simulink model "CubeSat_SDP_PD_Attitude"  (R2024b)
settings: Solver=FixedStepAuto  StartTime=0.0  StopTime=T_total  FixedStep=delta_t  MaxStep=delta_t  MinStep=delta_t
values from neighbouring files (symbols this model uses):
  Cross_section_area = 0.01    [initialize_satellite_simulation.m]
  finalAttitude = finalAttitude/norm(finalAttitude)    [initialize_satellite_simulation.m]
  J = diag([Jxx, Jxx, Jxx])    [calculateInertiaTensor.m]    (also in initialize_satellite_simulation.m = calculateInertiaTensor(mass, sideLength); solveSDPControl.m = reshape(u(9:17), 3, 3))
  J2 = J(2,2)    [cvx_sdp.m]
  k_d = 0.02    [initialize_satellite_simulation.m]
  k_p = 1.0    (= 1)    [initialize_satellite_simulation.m]
  mass = 1.33    [initialize_satellite_simulation.m]
undefined symbols (not defined in the file or in its folder): compute_drag
libraries: aerolibutil x6, aerolibgravity2 x1
settings Model: PauseTimes=0.2  PacingRate=1.100000  VariantFading=off  LastModifiedBy=shavykashyap
settings SolverCC: InitialStep=delta_t  ZeroCrossAlgorithm=Adaptive
settings DataIOCC: Refine=2
settings DebuggingCC: SignalInfNanChecking=error  MaskedZcDiagnostic=none  IgnoredZcDiagnostic=none  CheckMatrixSingularityMsg=error

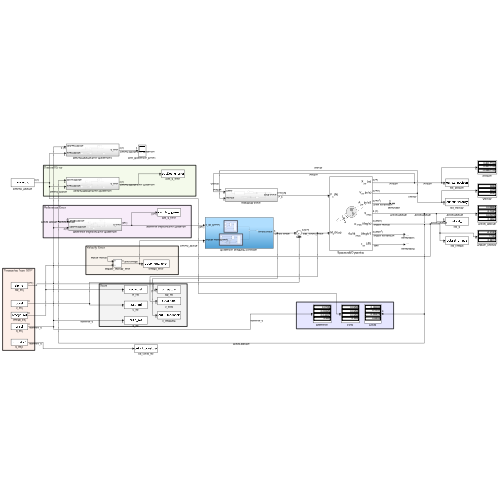
[thumbnail: Simulink's stored preview of the top-level diagram]
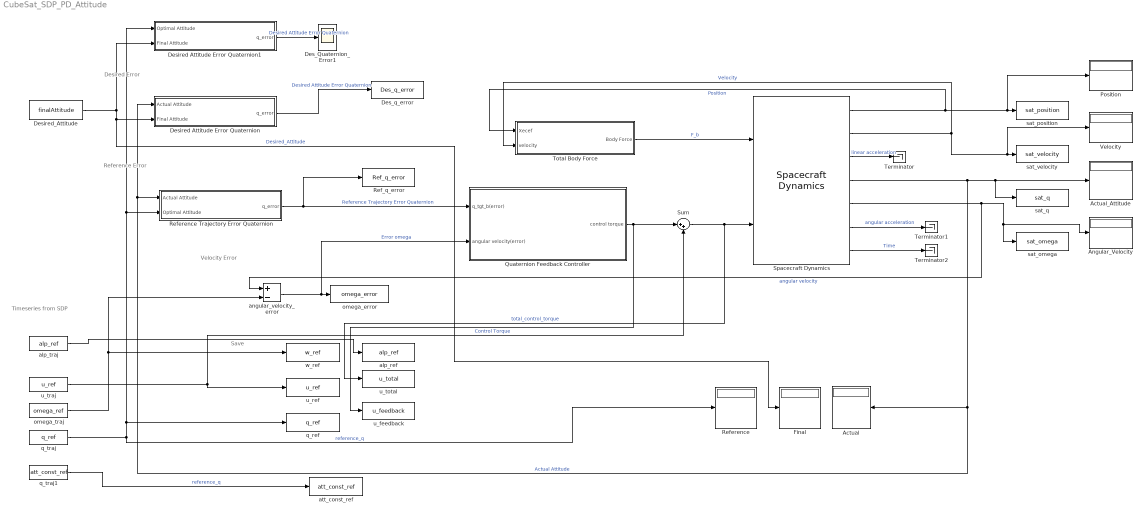
== system CubeSat_SDP_PD_Attitude ==
  note: Save
  note: Velocity Error
  note: Reference Error
  note: Timeseries from SDP
  note: Desired Error
  Actual : Display
  Actual_Attitude : Display
  "Angular_Velocity " : Display
  Des_Quaternion_Error1 : Scope
  Des_q_error : ToWorkspace  VariableName=Des_q_error  SaveFormat=Timeseries  SampleTime=-1
  Desired Attitude Error Quaternion : Subsystem
  Desired Attitude Error Quaternion1 : Subsystem
  Desired_Attitude : Constant  Value=finalAttitude
  Final : Display
  Position : Display
  "Quaternion Feedback Controller " : Subsystem
  Ref_q_error : ToWorkspace  VariableName=Ref_q_error  SaveFormat=Timeseries  SampleTime=-1
  Reference : Display
  Reference Trajectory Error Quaternion : Subsystem
  Spacecraft Dynamics : SpacecraftDynamics  outputAccel=on  mass=mass  inertia=J  stateFormatNum=ICRF state vector  inertialPosition=initialPosition  inertialVelocity=initialVelocity  attitude=initialAttitude  attitudeRate=initialAngularVelocity  outputAngAccel=on  gravityModel=Oblate ellipsoid (J2)  useDrag=on  useSRP=on
  Sum : Sum  Inputs=|++
  Terminator : Terminator
  Terminator1 : Terminator
  Terminator2 : Terminator
  "Total Body Force " : Subsystem
  Velocity : Display
  alp_ref : ToWorkspace  VariableName=alp_ref  SaveFormat=Timeseries  SampleTime=-1
  alp_traj : FromWorkspace  VariableName=alp_ref
  angular_velocity_error : Sum  Inputs=+-
  att_const_ref : ToWorkspace  VariableName=att_const_ref  SaveFormat=Timeseries  SampleTime=-1
  omega_error : ToWorkspace  VariableName=omega_error  SaveFormat=Timeseries  SampleTime=-1
  omega_traj : FromWorkspace  VariableName=omega_ref
  q_ref : ToWorkspace  VariableName=q_ref  SaveFormat=Timeseries  SampleTime=-1
  q_traj : FromWorkspace  VariableName=q_ref
  q_traj1 : FromWorkspace  VariableName=att_const_ref
  sat_omega : ToWorkspace  VariableName=sat_omega  SaveFormat=Timeseries  SampleTime=-1
  sat_position : ToWorkspace  VariableName=sat_position  SaveFormat=Timeseries  SampleTime=-1
  sat_q : ToWorkspace  VariableName=sat_q  SaveFormat=Timeseries  SampleTime=-1
  sat_velocity : ToWorkspace  VariableName=sat_velocity  SaveFormat=Timeseries  SampleTime=-1
  u_feedback : ToWorkspace  VariableName=u_feedback  SaveFormat=Timeseries  SampleTime=-1
  u_ref : ToWorkspace  VariableName=u_ref  SaveFormat=Timeseries  SampleTime=-1
  u_total : ToWorkspace  VariableName=u_total  SaveFormat=Timeseries  SampleTime=-1
  u_traj : FromWorkspace  VariableName=u_ref
  w_ref : ToWorkspace  VariableName=w_ref  SaveFormat=Timeseries  SampleTime=-1
  wires:
  Spacecraft Dynamics/1 -> "Total Body Force "/1(Xecef), Position/1, sat_position/1  "Position"
  Spacecraft Dynamics/2 -> Velocity/1, sat_velocity/1, "Total Body Force "/2(velocity)  "Velocity"
  Spacecraft Dynamics/4 -> Desired Attitude Error Quaternion/1(Actual Attitude), Reference Trajectory Error Quaternion/1(Actual Attitude), Actual/1, sat_q/1, Actual_Attitude/1  "Actual Attitude"
  Spacecraft Dynamics/5 -> angular_velocity_error/1, "Angular_Velocity "/1, sat_omega/1  "angular velocity"
  "Quaternion Feedback Controller "/1(control torque) -> Sum/1, u_feedback/1  "Control Torque"
  Desired_Attitude/1 -> Desired Attitude Error Quaternion/2(Final Attitude), Final/1, Desired Attitude Error Quaternion1/2(Final Attitude)  "Desired_Attitude"
  Spacecraft Dynamics/6 -> Terminator1/1  "angular acceleration"
  Spacecraft Dynamics/7 -> Terminator2/1  "Time"
  Spacecraft Dynamics/3 -> Terminator/1  "linear acceleration"
  "Total Body Force "/1(Body Force) -> Spacecraft Dynamics/1  "F_b"
  Sum/1 -> u_total/1, Spacecraft Dynamics/2  "total_control_torque"
  Reference Trajectory Error Quaternion/1(q_error) -> "Quaternion Feedback Controller "/1(q_tgt_b(error)), Ref_q_error/1  "Reference Trajectory Error Quaternion"
  angular_velocity_error/1 -> "Quaternion Feedback Controller "/2(angular velocity(error)), omega_error/1  "Error omega"
  Desired Attitude Error Quaternion/1(q_error) -> Des_q_error/1  "Desired Attitude Error Quaternion"
  u_traj/1 -> u_ref/1, Sum/2
  omega_traj/1 -> angular_velocity_error/2, w_ref/1
  q_traj/1 -> Reference/1, q_ref/1, Desired Attitude Error Quaternion1/1(Optimal Attitude), Reference Trajectory Error Quaternion/2(Optimal Attitude)  "reference_q"
  Desired Attitude Error Quaternion1/1(q_error) -> Des_Quaternion_Error1/1  "Desired Attitude Error Quaternion"
  alp_traj/1 -> alp_ref/1
  q_traj1/1 -> att_const_ref/1  "reference_q"

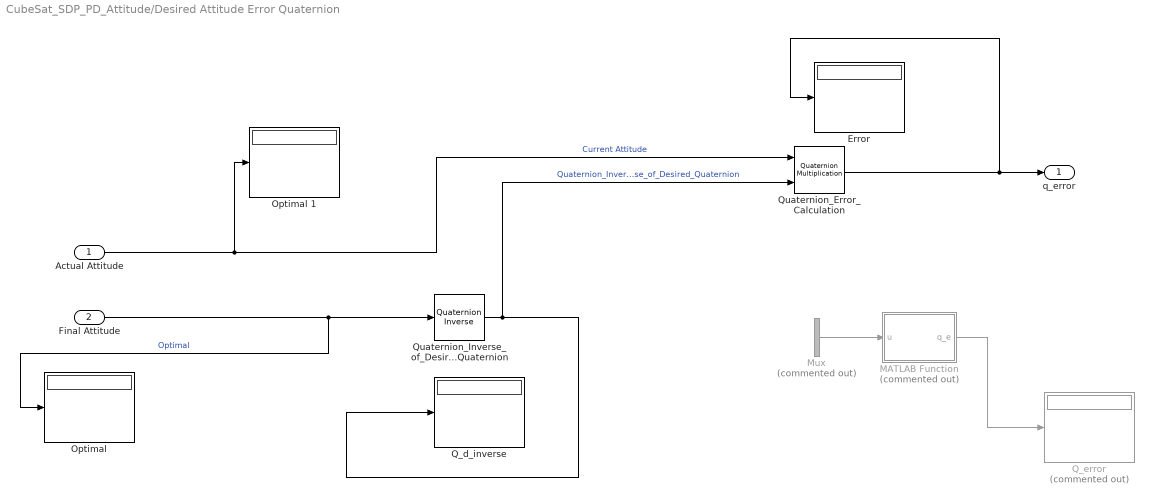
== system CubeSat_SDP_PD_Attitude/Desired Attitude Error Quaternion ==
  Actual Attitude : Inport
  Final Attitude : Inport  Port=2
  Error : Display
  MATLAB Function : MATLAB Function  Commented=on  TreatAsAtomicUnit=on
  Mux : Mux  Commented=on  Inputs=2
  "Optimal " : Display
  Optimal 1 : Display
  Q_d_inverse : Display
  Q_error : Display  Commented=on
  Quaternion_Error_Calculation : aerolibutil/Quaternion Multiplication
  Quaternion_Inverse_of_Desired_Quaternion : aerolibutil/Quaternion Inverse
  q_error : Outport
  wires:
  Actual Attitude/1 -> Optimal 1/1, Quaternion_Error_Calculation/1  "Current Attitude"
  Quaternion_Inverse_of_Desired_Quaternion/1 -> Quaternion_Error_Calculation/2, Q_d_inverse/1  "Quaternion_Inverse_of_Desired_Quaternion"
  Quaternion_Error_Calculation/1 -> q_error/1, Error/1
  Final Attitude/1 -> Quaternion_Inverse_of_Desired_Quaternion/1, "Optimal "/1  "Optimal"
  Mux/1 -> MATLAB Function/1(u)
  MATLAB Function/1(q_e) -> Q_error/1

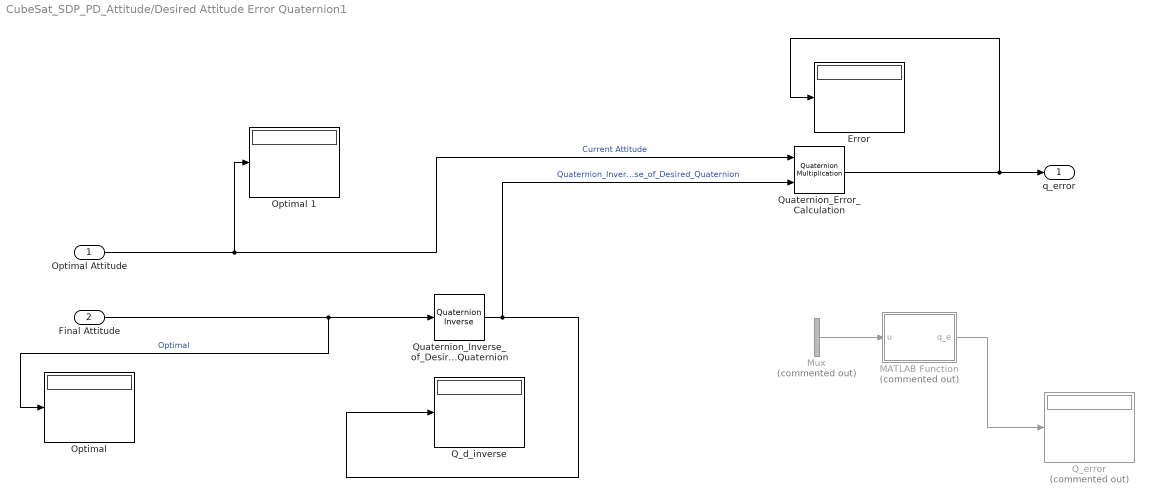
== system CubeSat_SDP_PD_Attitude/Desired Attitude Error Quaternion1 ==
  Optimal Attitude : Inport
  Final Attitude : Inport  Port=2
  Error : Display
  MATLAB Function : MATLAB Function  Commented=on  TreatAsAtomicUnit=on
  Mux : Mux  Commented=on  Inputs=2
  "Optimal " : Display
  Optimal 1 : Display
  Q_d_inverse : Display
  Q_error : Display  Commented=on
  Quaternion_Error_Calculation : aerolibutil/Quaternion Multiplication
  Quaternion_Inverse_of_Desired_Quaternion : aerolibutil/Quaternion Inverse
  q_error : Outport
  wires:
  Optimal Attitude/1 -> Optimal 1/1, Quaternion_Error_Calculation/1  "Current Attitude"
  Quaternion_Inverse_of_Desired_Quaternion/1 -> Quaternion_Error_Calculation/2, Q_d_inverse/1  "Quaternion_Inverse_of_Desired_Quaternion"
  Quaternion_Error_Calculation/1 -> q_error/1, Error/1
  Final Attitude/1 -> Quaternion_Inverse_of_Desired_Quaternion/1, "Optimal "/1  "Optimal"
  Mux/1 -> MATLAB Function/1(u)
  MATLAB Function/1(q_e) -> Q_error/1

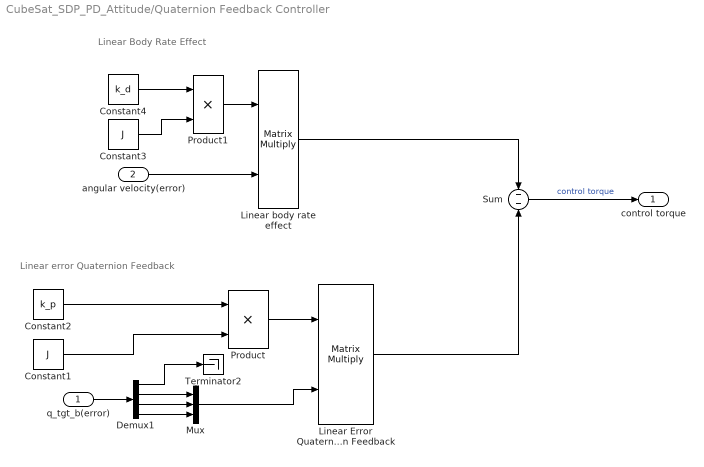
== system CubeSat_SDP_PD_Attitude/Quaternion Feedback Controller  ==
  note: Linear error Quaternion Feedback
  note: Linear Body Rate Effect
  q_tgt_b(error) : Inport
  angular velocity(error) : Inport  Port=2
  Constant1 : Constant  Value=J
  Constant2 : Constant  Value=k_p
  Constant3 : Constant  Value=J
  Constant4 : Constant  Value=k_d
  Demux1 : Demux
  Linear Error Quaternion Feedback : Product  Multiplication=Matrix(*)
  Linear body rate effect : Product  Multiplication=Matrix(*)
  Mux : Mux  Inputs=3
  Product : Product
  Product1 : Product
  Sum : Sum  Inputs=--
  Terminator2 : Terminator
  control torque : Outport
  wires:
  Linear body rate effect/1 -> Sum/1
  Mux/1 -> Linear Error Quaternion Feedback/2
  angular velocity(error)/1 -> Linear body rate effect/2
  Demux1/1 -> Terminator2/1
  Constant1/1 -> Product/2
  Linear Error Quaternion Feedback/1 -> Sum/2
  Demux1/4 -> Mux/3
  Constant2/1 -> Product/1
  Demux1/2 -> Mux/1
  Demux1/3 -> Mux/2
  Constant3/1 -> Product1/2
  q_tgt_b(error)/1 -> Demux1/1
  Sum/1 -> control torque/1  "control torque"
  Constant4/1 -> Product1/1
  Product/1 -> Linear Error Quaternion Feedback/1
  Product1/1 -> Linear body rate effect/1

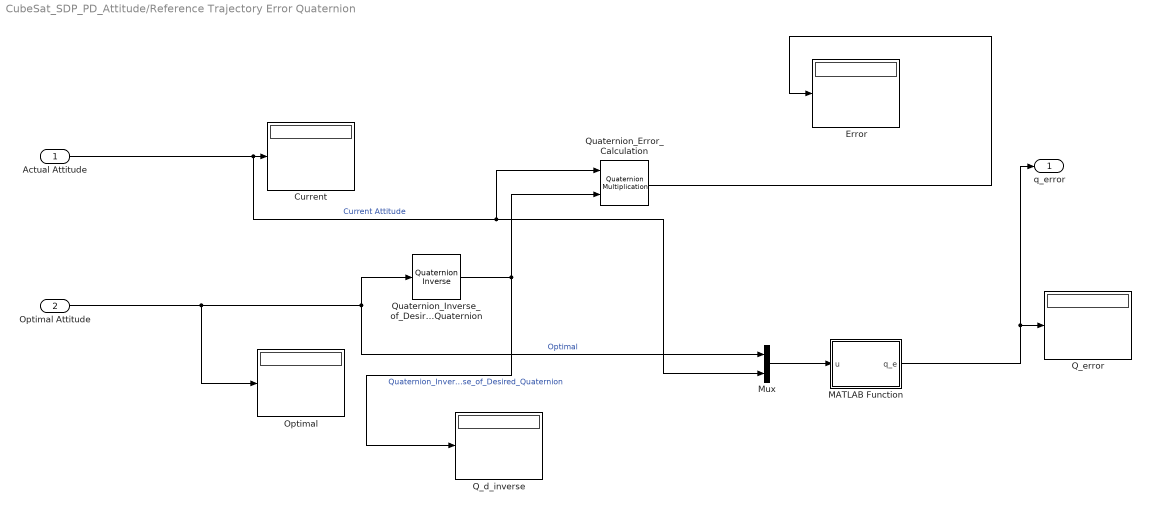
== system CubeSat_SDP_PD_Attitude/Reference Trajectory Error Quaternion ==
  Actual Attitude : Inport
  Optimal Attitude : Inport  Port=2
  Current : Display
  Error : Display
  MATLAB Function : MATLAB Function  TreatAsAtomicUnit=on
  Mux : Mux  Inputs=2
  "Optimal " : Display
  Q_d_inverse : Display
  Q_error : Display
  Quaternion_Error_Calculation : aerolibutil/Quaternion Multiplication
  Quaternion_Inverse_of_Desired_Quaternion : aerolibutil/Quaternion Inverse
  q_error : Outport
  wires:
  Actual Attitude/1 -> Mux/2, Quaternion_Error_Calculation/1, Current/1  "Current Attitude"
  Quaternion_Inverse_of_Desired_Quaternion/1 -> Q_d_inverse/1, Quaternion_Error_Calculation/2  "Quaternion_Inverse_of_Desired_Quaternion"
  Quaternion_Error_Calculation/1 -> Error/1
  Optimal Attitude/1 -> Mux/1, Quaternion_Inverse_of_Desired_Quaternion/1, "Optimal "/1  "Optimal"
  Mux/1 -> MATLAB Function/1(u)
  MATLAB Function/1(q_e) -> q_error/1, Q_error/1

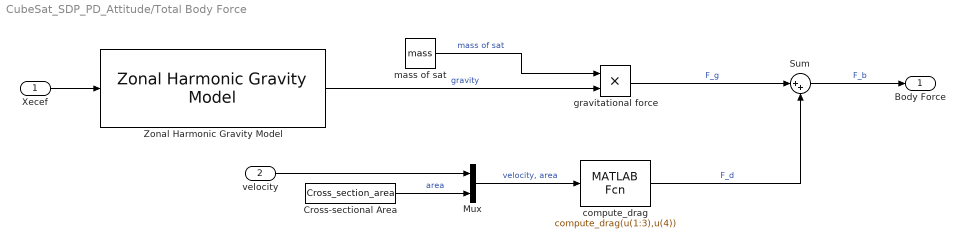
== system CubeSat_SDP_PD_Attitude/Total Body Force  ==
  Xecef : Inport
  velocity : Inport  Port=2
  Cross-sectional Area : Constant  Value=Cross_section_area
  Mux : Mux  Inputs=2
  Sum : Sum  Inputs=|++
  Zonal Harmonic Gravity Model : aerolibgravity2/Zonal Harmonic Gravity Model  units=Metric (MKS)  degree=4  action=Warning  ptype=Earth  R=6378136.3  GM=398600441500000  jvalue=[1.0826269e-03 -2.5323000e-06 -1.6204000e-06]
  compute_drag : MATLABFcn  MATLABFcn=compute_drag(u(1:3),u(4))
  gravitational force : Product
  mass of sat : Constant  Value=mass
  Body Force : Outport
  wires:
  mass of sat/1 -> gravitational force/1  "mass of sat"
  compute_drag/1 -> Sum/2  "F_d"
  Mux/1 -> compute_drag/1  "velocity, area"
  Cross-sectional Area/1 -> Mux/2  "area"
  gravitational force/1 -> Sum/1  "F_g"
  Zonal Harmonic Gravity Model/1 -> gravitational force/2  "gravity"
  Xecef/1 -> Zonal Harmonic Gravity Model/1
  Sum/1 -> Body Force/1  "F_b"
  velocity/1 -> Mux/1

== matlab function CubeSat_SDP_PD_Attitude/Desired Attitude Error Quaternion1/MATLAB Function ==
  data: u input; q_e output
function q_e = quaternionError(u)
    % quaternionError: Computes the quaternion error between two quaternions.
    % 
    % INPUTS:
    %   q_d - Desired quaternion (commanded attitude) [4x1 column vector]
    %   q   - Current quaternion (actual attitude) [4x1 column vector]
    %
    % OUTPUT:
    %   q_e - Quaternion error q_e = q * q_d^(-1) [4x1 column vector]

    % Extracting inputs that are in the form [a;
    %                                         b;
    %                                         c;
    %                                         d];
    q_d = u(1:4);
    q = u(5:8);

    % Correcting the dimensions for  
    % q_d = q_d';
    % q = q';

    % % Compute the conjugate of q_d (negate vector part, keep scalar unchanged)
    % q_d_conj = [q_d(1); -q_d(2:4)];

    % Compute the inverse of q_d (for unit quaternions, this is just its conjugate)
    q_d_inv = quatinv(q_d');    % Using the transpose , since the quatinv function requires [1x4] inputs 
    q_d_inv = q_d_inv';         % taking the transpose of the inverse to make the dimensions [4x1] which is required for the 

    % Compute quaternion error: q_e = q * q_d_inv (Hamilton product)
    % Quaternion multiplication formula:
    % Scalar part:  q_e(1) = q0 * p0 - (q_v • p_v)
    % Vector part:  q_e(2:4) = q0 * p_v + p0 * q_v - (q_v × p_v)
    q_e = [ q(1) * q_d_inv(1) - dot(q(2:4), q_d_inv(2:4));   % Scalar part
            q_d_inv(1) * q(2:4) + q(1) * q_d_inv(2:4) - cross(q(2:4), q_d_inv(2:4)) ]; % Vector part

    % q_e = q_e';
    % % Normalize quaternion error to ensure it remains a unit quaternion
    q_e = q_e / norm(q_e);
    % q_e = q_e';

end

== matlab function CubeSat_SDP_PD_Attitude/Desired Attitude Error Quaternion/MATLAB Function ==
  data: u input; q_e output
function q_e = quaternionError(u)
    % quaternionError: Computes the quaternion error between two quaternions.
    % 
    % INPUTS:
    %   q_d - Desired quaternion (commanded attitude) [4x1 column vector]
    %   q   - Current quaternion (actual attitude) [4x1 column vector]
    %
    % OUTPUT:
    %   q_e - Quaternion error q_e = q * q_d^(-1) [4x1 column vector]

    % Extracting inputs that are in the form [a;
    %                                         b;
    %                                         c;
    %                                         d];
    q_d = u(1:4);
    q = u(5:8);

    % Correcting the dimensions for  
    % q_d = q_d';
    % q = q';

    % % Compute the conjugate of q_d (negate vector part, keep scalar unchanged)
    % q_d_conj = [q_d(1); -q_d(2:4)];

    % Compute the inverse of q_d (for unit quaternions, this is just its conjugate)
    q_d_inv = quatinv(q_d');    % Using the transpose , since the quatinv function requires [1x4] inputs 
    q_d_inv = q_d_inv';         % taking the transpose of the inverse to make the dimensions [4x1] which is required for the 

    % Compute quaternion error: q_e = q * q_d_inv (Hamilton product)
    % Quaternion multiplication formula:
    % Scalar part:  q_e(1) = q0 * p0 - (q_v • p_v)
    % Vector part:  q_e(2:4) = q0 * p_v + p0 * q_v - (q_v × p_v)
    q_e = [ q(1) * q_d_inv(1) - dot(q(2:4), q_d_inv(2:4));   % Scalar part
            q_d_inv(1) * q(2:4) + q(1) * q_d_inv(2:4) - cross(q(2:4), q_d_inv(2:4)) ]; % Vector part

    % q_e = q_e';
    % % Normalize quaternion error to ensure it remains a unit quaternion
    q_e = q_e / norm(q_e);
    % q_e = q_e';

end

== matlab function CubeSat_SDP_PD_Attitude/Reference Trajectory Error Quaternion/MATLAB Function ==
  data: u input; q_e output
function q_e = quaternionError(u)
    % quaternionError: Computes the quaternion error between two quaternions.
    % 
    % INPUTS:
    %   q_d - Desired quaternion (commanded attitude) [4x1 column vector]
    %   q   - Current quaternion (actual attitude) [4x1 column vector]
    %
    % OUTPUT:
    %   q_e - Quaternion error q_e = q * q_d^(-1) [4x1 column vector]

    % Extracting inputs that are in the form [a;
    %                                         b;
    %                                         c;
    %                                         d];
    q_d = u(1:4);
    q = u(5:8);

    % Correcting the dimensions for  
    % q_d = q_d';
    % q = q';

    % % Compute the conjugate of q_d (negate vector part, keep scalar unchanged)
    % q_d_conj = [q_d(1); -q_d(2:4)];

    % Compute the inverse of q_d (for unit quaternions, this is just its conjugate)
    q_d_inv = (quatinv(q_d'))';    % Using the transpose , since the quatinv function requires [1x4] inputs 
    % q_d_inv = q_d_inv';         % taking the transpose of the inverse to make the dimensions [4x1] which is required for the 

    % Compute quaternion error: q_e = q * q_d_inv (Hamilton product)
    % Quaternion multiplication formula:
    % Scalar part:  q_e(1) = q0 * p0 - (q_v • p_v)
    % Vector part:  q_e(2:4) = q0 * p_v + p0 * q_v - (q_v × p_v)
    
    q_e = [ q(1) * q_d_inv(1) - dot(q(2:4), q_d_inv(2:4));   % Scalar part
            q_d_inv(1) * q(2:4) + q(1) * q_d_inv(2:4) - cross(q(2:4), q_d_inv(2:4)) ]; % Vector part

    % q_e = q_e';
    % % Normalize quaternion error to ensure it remains a unit quaternion
    q_e = q_e / norm(q_e);
    % q_e = q_e';

end
